simulink model "delay_track_fshift_sim"  (R2019a)
settings: Solver=VariableStepAuto  StartTime=0.0  StopTime=500000 / (fs_ghz * 1e9)  RelTol=1e-3
undefined symbols (not defined in the file or in its folder): fdesignblkfcn, fs_ghz, gcbh
libraries: dspmtrx3 x5, dspxfrm3 x2, simulink x1
(part 4 of 7)

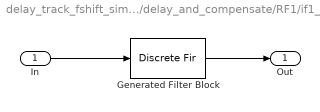
== system delay_track_fshift_sim/delay_and_compensate/RF1/if1_filt ==
  In : Inport
  Generated Filter Block : DiscreteFir  Tag=BlockMethodSubSystem  Coefficients=[3.4793427262309392e-05 5.44930009021886444e-05 7.67230161640516311e-06 -4.90795005220614759e-05 -5.00251028970550559e-05 3.70846460305349548e-05 0.000185516672775070751 0.000317032928598762903 0.000341105037848429924 0.000206892118281761336 -5.9982989554209261e-05 -0.00035835848219169399 -0.000554209791067096871 -0.000546424234637173838 -0.000322177302977984053 2.93739649481302108e-05 0.000356381821158042783 0.000519422639733093609 0.00046361346106178243 0.000247243728928788116 7.92728804893087412e-06 -0.000118081345883584777 -7.88950157538884783e-05 5.75688027569752479e-05 0.000141712690478337674 3.77750198706143262e-05 -0.000276568495203525632 -0.000668912990085496467 -0.000903738265255738123 -0.000769188989900463217 -0.00021303589019783947 0.00059276752876120508 0.0013076699574674595 0.00158225970267628644 0.00124332636612618807 0.000401936724042846927 -0.000583853274264716686 -0.0012828553743162276 -0.00141320627367778743 -0.000990709352046571573 -0.000314483979567378876 0.000209792073580028368 0.000313124752641961686 3.08463553168273751e-05 -0.000312373746314054135 -0.000304867191156925961 0.000271778742936110173 0.00125244013449563279 0.00211846105628497351 0.00225805885597095413 0.00132849230167535236 -0.000484833720890234441 -0.00247933253867256478 -0.00374289042557195183 -0.00361502034861769595 -0.00205606339824033861 0.000290044200907173971 0.00239662437168007168 0.00337365186289025022 0.00292739399430451842 0.00150020025231294976 -6.36017918822378866e-18 -0.000738326658563957577 -0.000453670339125073927 0.00037888479783360307 0.000840766559234820948 0.000168800663146957306 -0.00168543845951289197 -0.00388736543918710925 -0.00509000733117947069 -0.00418140243003806665 -0.00100476977188203895 0.00337827434859150084 0.00708734047659677086 0.0083279816830413439 0.00634012755765562142 0.0018656385794821376 -0.00315769037916522168 -0.00655307169649532381 -0.00701694091191249879 -0.00477678565903475426 -0.00141220096638349098 0.00108388163463838554 0.00148589294526874235 7.41281752089690974e-05 -0.00153036279516057167 -0.00138811672277394985 0.00144157161336614346 0.006073793761855119 0.0100230885977322694 0.010467312075857188 0.00591805676699343804 -0.0026412871020297015 -0.0118779818872822816 -0.0175698717877994758 -0.0167246564928610029 -0.00924463827339409502 0.00181858083060367133 0.0116645454252521132 0.0161411590251471539 0.0138799773897710418 0.00697606106549465959 -0.000237456095176756326 -0.00371782099366803299 -0.00215465708063087387 0.0021177836486976063 0.00441048368650510513 0.000615873708072903875 -0.00979343604670627164 -0.0225122198907671926 -0.0299195634191074811 -0.0249287865070437625 -0.00534356894264965444 0.0236520837180365755 0.0505541287942229065 0.0621522888704108267 0.0498219385529098113 0.0145125250941886327 -0.0322341147478608647 -0.0722020458178861263 -0.0879862767412204066 -0.0708260794321600856 -0.0251568832118651796 0.0324355195625202278 0.0796865267172618963 0.0978632747395140473 0.0796865267172618963 0.0324355195625202278 -0.0251568832118651796 -0.0708260794321600856 -0.0879862767412204066 -0.0722020458178861263 -0.0322341147478608647 0.0145125250941886327 0.0498219385529098113 0.0621522888704108267 0.0505541287942229065 0.0236520837180365755 -0.00534356894264965444 -0.0249287865070437625 -0.0299195634191074811 -0.0225122198907671926 -0.00979343604670627164 0.000615873708072903875 0.00441048368650510513 0.0021177836486976063 -0.00215465708063087387 -0.00371782099366803299 -0.000237456095176756326 0.00697606106549465959 0.0138799773897710418 0.0161411590251471539 0.0116645454252521132 0.00181858083060367133 -0.00924463827339409502 -0.0167246564928610029 -0.0175698717877994758 -0.0118779818872822816 -0.0026412871020297015 0.00591805676699343804 0.010467312075857188 0.0100230885977322694 0.006073793761855119 0.00144157161336614346 -0.00138811672277394985 -0.00153036279516057167 7.41281752089690974e-05 0.00148589294526874235 0.00108388163463838554 -0.00141220096638349098 ...(+1940 chars)]  InputProcessing=Columns as channels (frame based)
  Out : Outport
  wires:
  Generated Filter Block/1 -> Out/1
  In/1 -> Generated Filter Block/1
